simulink model "xtrlmod"  (Simulink 3.00)
settings: Solver=ode45  StartTime=0.0  StopTime=360.0  RelTol=1e-3
settings Model: ExtModeTrigMode=normal  ExtModeArmWhenConnect=on

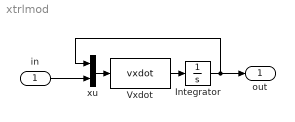
== system xtrlmod ==
  in : Inport  Port=1  PortWidth=-1  SampleTime=-1  DataType=auto
      settings: SignalType=auto
  Integrator : Integrator  ExternalReset=none  InitialConditionSource=internal  InitialCondition=0  LimitOutput=off  UpperSaturationLimit=inf  LowerSaturationLimit=-inf  ShowSaturationPort=off  ShowStatePort=off  AbsoluteTolerance=auto
  Vxdot : MATLABFcn  MATLABFcn=vxdot  OutputWidth=12  OutputSignalType=real
  xu : Mux  Inputs=[12 26]
  out : Outport  Port=1
  wires:
  in/1 -> xu/2
  xu/1 -> Vxdot/1
  Integrator/1 -> xu/1, out/1
  Vxdot/1 -> Integrator/1
